simulink model "wingrockRBF"  (R2022b)
settings: Solver=VariableStepAuto  StartTime=0.0  StopTime=Tf  RelTol=1e-3
undefined symbols (not defined in the file): A, B
libraries: dspsigattribs x4, slctrlblks x1
settings Model: Creator=The MathWorks, Inc.  LastModifiedBy=Claudia Yasar
settings SolverCC: MaxZcPerStep=1
settings DataIOCC: ReturnWorkspaceOutputs=off
settings DebuggingCC: UnconnectedInputMsg=warning  UnconnectedOutputMsg=warning  UnconnectedLineMsg=warning
settings ModelReferenceCC: EnableRefExpFcnMdlSchedulingChecks=on
settings RTWCC: DLArmComputeVersion=19.05

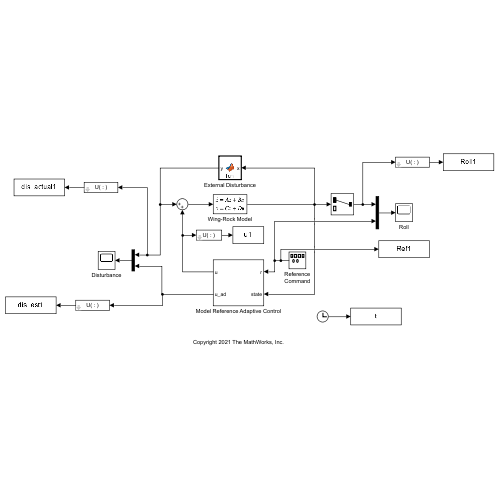
[thumbnail: Simulink's stored preview of the top-level diagram]
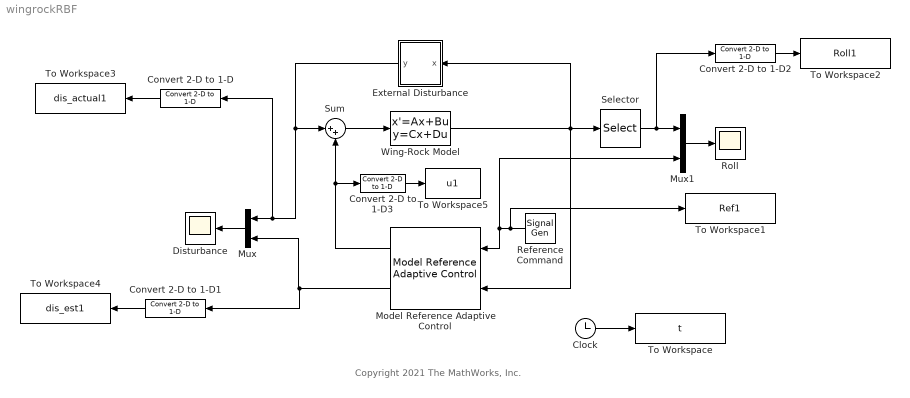
== system wingrockRBF ==
  note: Copyright 2021 The MathWorks, Inc.
  Clock : Clock
  Convert 2-D to 1-D{,1..3} (4 alike) : dspsigattribs/Convert 2-D to 1-D
  Disturbance : Scope
  External Disturbance : MATLAB Function  TreatAsAtomicUnit=on
  Model Reference Adaptive Control : slctrlblks/Model Reference Adaptive Control  selectType=Direct  A=A  B=B  Ahat=0  ALrEnable=on  gamma_a=1  ALrEnableMod=on  Bhat=1  BLrEnable=on  gamma_b=1  BLrEnableMod=on  externalKtauEnable=off  k_tau=-1  estParamOutput=off  Am=Am  Bm=Bm  kx=Kx  FBLrEnable=off  gamma_kx=1  FBLrEnableMod=on  kr=Kr  FFLrEnable=off  gamma_kr=1  FFLrEnableMod=on  AdaptEnable=on  gamma=gamma_w  WLrEnableMod=off  Q=Q  FeatureTypeOptions=Radial Basis Function  nCen=N  cSpanMin=cen_min  cSpanMax=cen_max  cSig=bandwidth  adaptiveCntrlOutport=on  modChoice=None  sigma_val=0.1
  Mux : Mux  Inputs=2
  Mux1 : Mux  Inputs=2
  Reference Command : SignalGenerator  WaveForm=square  Frequency=0.5  Units=rad/sec
  Roll : Scope
  Selector : Selector  InputPortWidth=2  IndexOptions=Index vector (dialog)  Indices=1  OutputSizes=1
  Sum : Sum  Inputs=|++
  To Workspace : ToWorkspace  VariableName=t  SampleTime=-1
      settings: Save2DSignal=2-D array (concatenate along first dimension)
  To Workspace1 : ToWorkspace  VariableName=Ref1  SampleTime=-1
      settings: Save2DSignal=2-D array (concatenate along first dimension)
  To Workspace2 : ToWorkspace  VariableName=Roll1  SampleTime=-1
      settings: Save2DSignal=2-D array (concatenate along first dimension)
  To Workspace3 : ToWorkspace  VariableName=dis_actual1  SampleTime=-1
      settings: Save2DSignal=2-D array (concatenate along first dimension)
  To Workspace4 : ToWorkspace  VariableName=dis_est1  SampleTime=-1
      settings: Save2DSignal=2-D array (concatenate along first dimension)
  To Workspace5 : ToWorkspace  VariableName=u1  SampleTime=-1
  Wing-Rock Model : StateSpace  A=[0 1;0 0]  B=[0;1]  C=eye(2)  D=[0;0]  InitialCondition=0
  wires:
  Sum/1 -> Wing-Rock Model/1
  Model Reference Adaptive Control/1 -> Convert 2-D to 1-D3/1, Sum/2
  Wing-Rock Model/1 -> Model Reference Adaptive Control/2, Selector/1, External Disturbance/1(x)
  Mux/1 -> Disturbance/1
  Mux1/1 -> Roll/1
  Convert 2-D to 1-D/1 -> To Workspace3/1
  External Disturbance/1(y) -> Sum/1, Convert 2-D to 1-D/1, Mux/1
  Reference Command/1 -> To Workspace1/1, Model Reference Adaptive Control/1, Mux1/2
  Clock/1 -> To Workspace/1
  Convert 2-D to 1-D2/1 -> To Workspace2/1
  Selector/1 -> Convert 2-D to 1-D2/1, Mux1/1
  Convert 2-D to 1-D3/1 -> To Workspace5/1
  Convert 2-D to 1-D1/1 -> To Workspace4/1
  Model Reference Adaptive Control/2 -> Convert 2-D to 1-D1/1, Mux/2

== matlab function wingrockRBF/External Disturbance ==
  data: y output; x input
function y = fcn(x)

phi = [1 x(1) x(2) abs(x(1))*x(2) abs(x(2))*x(2) x(1)^3];

w = [1 0.2314 0.6918 0.6245 0.1 0.214];

u = w*phi';

y = u;
